simulink model "observadores"  (R2021a)
settings: Solver=VariableStepAuto  StartTime=0.0  StopTime=3  FixedStep=0.01  RelTol=1e-3
settings Model: Creator=facun  LastModifiedBy=facun

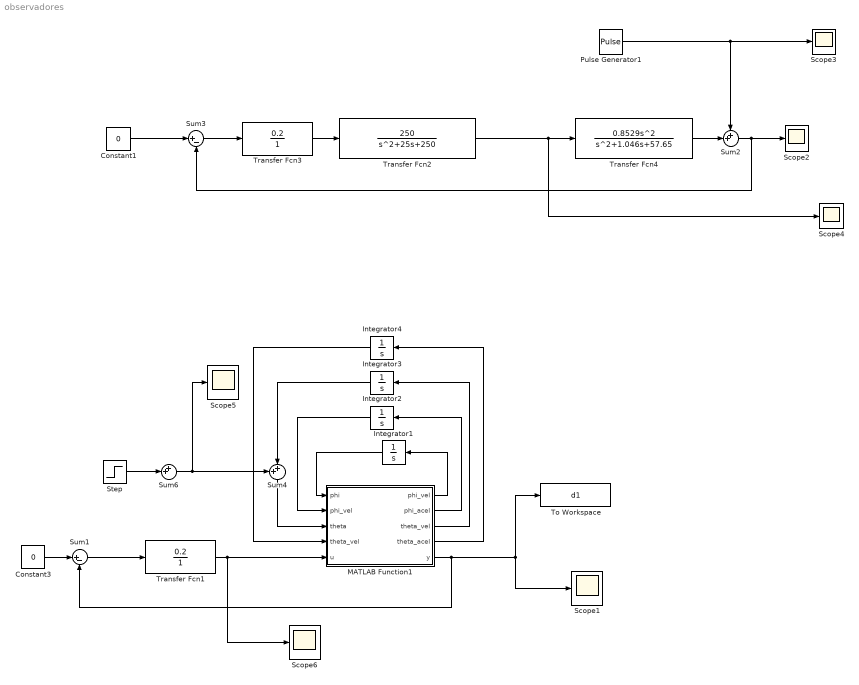
== system observadores ==
  Constant1 : Constant  Value=0
  Constant3 : Constant  Value=0
  Integrator{1..4} (4 alike) : Integrator
  MATLAB Function1 : MATLAB Function  TreatAsAtomicUnit=on
  Pulse Generator1 : DiscretePulseGenerator  PulseType=Time based  Amplitude=10  Period=10  PulseWidth=0.5  PhaseDelay=0.5
  Scope{1..6} (6 alike) : Scope
  Step : Step  Time=0.1  After=50  SampleTime=0
  Sum1 : Sum  Inputs=|+-
  Sum2 : Sum  Inputs=++|
  Sum3 : Sum  Inputs=|+-
  Sum4 : Sum  Inputs=++|
  Sum6 : Sum  Inputs=++|
  To Workspace : ToWorkspace  VariableName=d1  SampleTime=-1
      settings: Save2DSignal=2-D array (concatenate along first dimension)
  Transfer Fcn1 : TransferFcn  Numerator=[0.2]  Denominator=[1]
  Transfer Fcn2 : TransferFcn  Numerator=[250]  Denominator=[1 25 250]
  Transfer Fcn3 : TransferFcn  Numerator=[0.2]  Denominator=[1]
  Transfer Fcn4 : TransferFcn  Numerator=[0.8529 0 0]  Denominator=[1 1.046 57.65]
  wires:
  Pulse Generator1/1 -> Scope3/1, Sum2/1
  Constant1/1 -> Sum3/1
  Transfer Fcn3/1 -> Transfer Fcn2/1
  Sum3/1 -> Transfer Fcn3/1
  Sum2/1 -> Sum3/2, Scope2/1
  Transfer Fcn2/1 -> Scope4/1, Transfer Fcn4/1
  Transfer Fcn4/1 -> Sum2/2
  MATLAB Function1/1(phi_vel) -> Integrator1/1
  MATLAB Function1/2(phi_acel) -> Integrator2/1
  Integrator2/1 -> MATLAB Function1/2("phi_vel ")
  MATLAB Function1/3(theta_vel) -> Integrator3/1
  MATLAB Function1/5(y) -> To Workspace/1, Scope1/1, Sum1/2
  Transfer Fcn1/1 -> Scope6/1, MATLAB Function1/5(u)
  Integrator1/1 -> MATLAB Function1/1(phi)
  Sum1/1 -> Transfer Fcn1/1
  Constant3/1 -> Sum1/1
  Integrator4/1 -> MATLAB Function1/4("theta_vel ")
  MATLAB Function1/4(theta_acel) -> Integrator4/1
  Integrator3/1 -> Sum4/2
  Sum4/1 -> MATLAB Function1/3(theta)
  Sum6/1 -> Sum4/1, Scope5/1
  Step/1 -> Sum6/2

== matlab function observadores/MATLAB Function1 ==
  data: phi input; phi_vel input; theta input; theta_vel input; u input; phi_vel output; phi_acel output; theta_vel output; theta_acel output; y output
function [phi_vel,phi_acel,theta_vel,theta_acel,y] = fcn(phi,phi_vel,theta,theta_vel,u)

a = 250;
b = 25;
c = a;
d = 0.8529;
e = 1.046;
f = 57.65;

phi_acel = a * u - b * phi_vel - c * phi;
theta_acel = d * phi_acel - e * theta_vel - f * theta;
y=theta;
